simulink model "Quadrotor_eliminated_v2"  (R2020a)
settings: Solver=FixedStepAuto  StartTime=0.0  StopTime=options.T_train  FixedStep=options.dt  RelTol=1e-6
undefined symbols (not defined in the file or in its folder): options, Quad
libraries: neural x179, simulink x2
(part 5 of 10)

== system Quadrotor_eliminated_v2/NN/Layer 2/Delays 1 ==
  "p{2}" : Inport  PortDimensions=50
      mask Display: e = 0.06;c1 = [120 230 180]/255;c2 = ([120 230 180]+0)/(256+128);c3 = ([120 230 180]+128)/(256+128);patch([0 1 1 0],[0 0 1 1],c1);patch([0 1 1 1-e 1-e 0+e],[0 0 1 1-e 0+e 0+e],c2);patch([0 0 1 1-e 0+e 0+e],[0 1 1 1-e 1-e 0+e],c3);plot([0 1 1 0 0],[0 0 1 1 0]);
  mux : Mux  Inputs=1
      mask Display: e = 0.06;c1 = [120 150 230]/255;c2 = ([120 150 230]+0)/383;c3 = ([120 150 230]+128)/383;patch([0 1 1 0],[0 0 1 1],c1);patch([0 1 1 1-e 1-e 0+e],[0 0 1 1-e 0+e 0+e],c2);patch([0 0 1 1-e 0+e 0+e],[0 1 1 1-e 1-e 0+e],c3);plot([0 1 1 0 0],[0 0 1 1 0]);disp('Mux')
  "pd{2,1}" : Outport
      mask Display: e = 0.06;c1 = [120 230 180]/255;c2 = ([120 230 180]+0)/(256+128);c3 = ([120 230 180]+128)/(256+128);patch([0 1 1 0],[0 0 1 1],c1);patch([0 1 1 1-e 1-e 0+e],[0 0 1 1-e 0+e 0+e],c2);patch([0 0 1 1-e 0+e 0+e],[0 1 1 1-e 1-e 0+e],c3);plot([0 1 1 0 0],[0 0 1 1 0]);
  wires:
  "p{2}"/1 -> mux/1
  mux/1 -> "pd{2,1}"/1

== system Quadrotor_eliminated_v2/NN/Layer 2/LW{2,1} ==
  "ad{2,1}" : Inport  PortDimensions=50
      mask Display: e = 0.06;c1 = [120 230 180]/255;c2 = ([120 230 180]+0)/(256+128);c3 = ([120 230 180]+128)/(256+128);patch([0 1 1 0],[0 0 1 1],c1);patch([0 1 1 1-e 1-e 0+e],[0 0 1 1-e 0+e 0+e],c2);patch([0 0 1 1-e 0+e 0+e],[0 1 1 1-e 1-e 0+e],c3);plot([0 1 1 0 0],[0 0 1 1 0]);
  "IW{2,1}(1,:)'" : Constant  Value=[-0.3770749648986442270626184836146421730518341064453125;0.49419295175803146236148677417077124118804931640625;0.268525847491733582472761554527096450328826904296875;-1.909072408150881638988494160003028810024261474609375;0.71079573518007943544461113560828380286693572998046875;1.0910744222626533872499976496328599750995635986328125;-2.777749591094742953600871260277926921844482421875;-0.41521756252196950764954408441553823649883270263671875;0.0217747390108936796082605980018342961557209491729736328125;0.90040566650762954292730455563287250697612762451171875;-0.47920768443152839122234354363172315061092376708984375;-1.9101507442203544684389271424151957035064697265625;0.184768543321555622771512616964173503220081329345703125;0.194686844977042416982015993198729120194911956787109375;-0.3752613339416175364249284029938280582427978515625;-1.32896234468996876643132054596208035945892333984375;0.00953244374435228969399958032227004878222942352294921875;-0.282819860640611542290656643672264181077480316162109375;0.308268833807189335249887562895310111343860626220703125;-1.7686120089152475021165855650906451046466827392578125;2.272391307368064605753943396848626434803009033203125;-2.238801038566336831792114026029594242572784423828125;3.346582886223399722069871131679974496364593505859375;-0.88962659270552302270829159169807098805904388427734375;4.40677940570399773179133262601681053638458251953125;-0.2196973559701187739268135601378162391483783721923828125;-0.775392562457375422724226154969073832035064697265625;1.7604243446106748738344549565226770937442779541015625;1.5879078296333759556802078805048950016498565673828125;2.500769649404443129014907754026353359222412109375;3.880701197715260786225144329364411532878875732421875;0.142857236421507327595037395440158434212207794189453125;0.250827449428068727232954415740096010267734527587890625;1.05829790296190129339493068982847034931182861328125;0.59420297513869957395371557140606455504894256591796875;-1.9185354242740484398410671929013915359973907470703125;0.243084015573275358246263522232766263186931610107421875;-0.2998316457203282769938823548727668821811676025390625;-0.335818106926641546383649483686895109713077545166015625;0.0215143757209804963037580449736196896992623805999755859375;-0.54308832995387168462997351525700651109218597412109375;-1.0277285412017977961340875481255352497100830078125;-0.75434976423822064361957018263638019561767578125;0.7536334676355498363164997499552555382251739501953125;-0.1460991595714455637544659794002654962241649627685546875;-1.385288355222385359155623518745414912700653076171875;-3.2200800123955009013343442347832024097442626953125;-0.361848281263478732672211890530888922512531280517578125;0.1835251775307588928409785467010806314647197723388671875;0.38468780224319532035082147558568976819515228271484375]
      mask Display: e = 0.06;c1 = [120 150 230]/255;c2 = ([120 150 230]+0)/383;c3 = ([120 150 230]+128)/383;patch([0 1 1 0],[0 0 1 1],c1);patch([0 1 1 1-e 1-e 0+e],[0 0 1 1-e 0+e 0+e],c2);patch([0 0 1 1-e 0+e 0+e],[0 1 1 1-e 1-e 0+e],c3);plot([0 1 1 0 0],[0 0 1 1 0]);disp('weights');
  "IW{2,1}(2,:)'" : Constant  Value=[-0.6504497882364479455219452574965544044971466064453125;-0.2509436690938093850178347565815784037113189697265625;0.4113023030317661810073559536249376833438873291015625;-0.7761958482427087080424144005519337952136993408203125;0.199862762148222239400041644330485723912715911865234375;1.238336301499751268551108296378515660762786865234375;-2.455196469571485184957282399409450590610504150390625;0.08879563405870470604863697872133343480527400970458984375;-0.044403950219580871905389329867830383591353893280029296875;-1.2254644153788267768590003470308147370815277099609375;-0.91249641838621275979903657571412622928619384765625;-1.6196605249767281886619230135693214833736419677734375;0.74939773332802095406890430240309797227382659912109375;-0.63273524287853211145460363695747219026088714599609375;0.335299346622573712917159127755439840257167816162109375;1.7409296294815657102361683428171090781688690185546875;0.033843629506687671060216615614990587346255779266357421875;0.03207113846562124892525247332741855643689632415771484375;-0.260697643074277840558039542884216643869876861572265625;1.333555365978469797738625857164151966571807861328125;0.90374956704706133070459372902405448257923126220703125;-1.3892648340493771730308480982785113155841827392578125;1.5837025221033964594852250229450874030590057373046875;0.04693216881807589502262345604322035796940326690673828125;-4.00823867124373212078580763773061335086822509765625;0.51613112724687615351371050564921461045742034912109375;-0.0752672995684040835318029394329641945660114288330078125;-0.404503932865377946459517488619894720613956451416015625;0.9531031434354086950833107039215974509716033935546875;-0.5816847408341756509031483801663853228092193603515625;-1.104286169027709707535223060403950512409210205078125;1.0001200686984799137491108922404237091541290283203125;0.1835246472099729686533464700914919376373291015625;-0.28924059189118722645872594512184150516986846923828125;0.67843248076150197700684429946704767644405364990234375;-0.9173248522579882102689907696912996470928192138671875;-0.04185157138806505638939370328444056212902069091796875;-0.1681491751664594691551002370033529587090015411376953125;-0.344096144071270815256724517894326709210872650146484375;0.07410003550236059222111606459293398074805736541748046875;1.6085717979429936530522127213771454989910125732421875;0.63161572346059091653813766242819838225841522216796875;-0.38926216470056973495417196318157948553562164306640625;0.18652793546433621418856318996404297649860382080078125;-0.444026094858502917706033485956140793859958648681640625;-1.7593356490836102867802992477663792669773101806640625;-0.72154129771463881848347909908625297248363494873046875;-0.275270172576594973623542728091706521809101104736328125;-0.210165637309702557633528385849785991013050079345703125;-0.2351376060953877800141498255470651201903820037841796875]
      mask Display: e = 0.06;c1 = [120 150 230]/255;c2 = ([120 150 230]+0)/383;c3 = ([120 150 230]+128)/383;patch([0 1 1 0],[0 0 1 1],c1);patch([0 1 1 1-e 1-e 0+e],[0 0 1 1-e 0+e 0+e],c2);patch([0 0 1 1-e 0+e 0+e],[0 1 1 1-e 1-e 0+e],c3);plot([0 1 1 0 0],[0 0 1 1 0]);disp('weights');
  Mux : Mux  Inputs=2
      mask Display: e = 0.06;c1 = [120 150 230]/255;c2 = ([120 150 230]+0)/383;c3 = ([120 150 230]+128)/383;patch([0 1 1 0],[0 0 1 1],c1);patch([0 1 1 1-e 1-e 0+e],[0 0 1 1-e 0+e 0+e],c2);patch([0 0 1 1-e 0+e 0+e],[0 1 1 1-e 1-e 0+e],c3);plot([0 1 1 0 0],[0 0 1 1 0]);disp('Mux');
  dotprod1 : neural/Weight Functions/dotprod
  dotprod2 : neural/Weight Functions/dotprod
  "lz{2,1}" : Outport
      mask Display: e = 0.06;c1 = [120 230 180]/255;c2 = ([120 230 180]+0)/(256+128);c3 = ([120 230 180]+128)/(256+128);patch([0 1 1 0],[0 0 1 1],c1);patch([0 1 1 1-e 1-e 0+e],[0 0 1 1-e 0+e 0+e],c2);patch([0 0 1 1-e 0+e 0+e],[0 1 1 1-e 1-e 0+e],c3);plot([0 1 1 0 0],[0 0 1 1 0]);
  wires:
  "IW{2,1}(1,:)'"/1 -> dotprod1/1
  "ad{2,1}"/1 -> dotprod1/2, dotprod2/2
  dotprod1/1 -> Mux/1
  "IW{2,1}(2,:)'"/1 -> dotprod2/1
  dotprod2/1 -> Mux/2
  Mux/1 -> "lz{2,1}"/1

== system Quadrotor_eliminated_v2/NN_cex_1/Layer 1/Delays 1 ==
  "p{1}" : Inport  PortDimensions=15
      mask Display: e = 0.06;c1 = [120 230 180]/255;c2 = ([120 230 180]+0)/(256+128);c3 = ([120 230 180]+128)/(256+128);patch([0 1 1 0],[0 0 1 1],c1);patch([0 1 1 1-e 1-e 0+e],[0 0 1 1-e 0+e 0+e],c2);patch([0 0 1 1-e 0+e 0+e],[0 1 1 1-e 1-e 0+e],c3);plot([0 1 1 0 0],[0 0 1 1 0]);
  mux : Mux  Inputs=1
      mask Display: e = 0.06;c1 = [120 150 230]/255;c2 = ([120 150 230]+0)/383;c3 = ([120 150 230]+128)/383;patch([0 1 1 0],[0 0 1 1],c1);patch([0 1 1 1-e 1-e 0+e],[0 0 1 1-e 0+e 0+e],c2);patch([0 0 1 1-e 0+e 0+e],[0 1 1 1-e 1-e 0+e],c3);plot([0 1 1 0 0],[0 0 1 1 0]);disp('Mux')
  "pd{1,1}" : Outport
      mask Display: e = 0.06;c1 = [120 230 180]/255;c2 = ([120 230 180]+0)/(256+128);c3 = ([120 230 180]+128)/(256+128);patch([0 1 1 0],[0 0 1 1],c1);patch([0 1 1 1-e 1-e 0+e],[0 0 1 1-e 0+e 0+e],c2);patch([0 0 1 1-e 0+e 0+e],[0 1 1 1-e 1-e 0+e],c3);plot([0 1 1 0 0],[0 0 1 1 0]);
  wires:
  "p{1}"/1 -> mux/1
  mux/1 -> "pd{1,1}"/1
